simulink model "Alpha_beta_V"  (R2013a)
settings: Solver=ode45  StartTime=0.0  StopTime=10.0  RelTol=1e-3
settings Model: Creator=Ibrahim_B92  LastModifiedBy=Ibrahim_B92

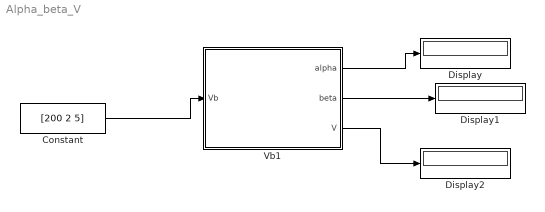
== system Alpha_beta_V ==
  Constant : Constant  Value=[200 2 5]
  Display : Display
  Display1 : Display
  Display2 : Display
  Vb1 : Subsystem
  wires:
  Constant/1 -> Vb1/1(Vb)
  Vb1/1(alpha) -> Display/1
  Vb1/2(beta) -> Display1/1
  Vb1/3(V) -> Display2/1

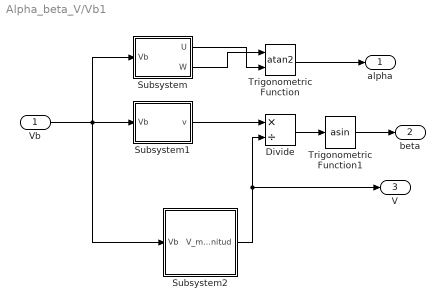
== system Alpha_beta_V/Vb1 ==
  Vb : Inport
  Divide : Product  Inputs=*/
  Subsystem : Subsystem
  Subsystem1 : Subsystem
  Subsystem2 : Subsystem
  Trigonometric Function : Trigonometry  Operator=atan2
  Trigonometric Function1 : Trigonometry  Operator=asin
  alpha : Outport
  beta : Outport  Port=2
  V : Outport  Port=3
  wires:
  Subsystem2/1(V_magnitud) -> Divide/2, V/1
  Subsystem/2(W) -> Trigonometric Function/1
  Subsystem/1(U) -> Trigonometric Function/2
  Trigonometric Function/1 -> alpha/1
  Subsystem1/1(v) -> Divide/1
  Divide/1 -> Trigonometric Function1/1
  Trigonometric Function1/1 -> beta/1
  Vb/1 -> Subsystem2/1(Vb), Subsystem/1(Vb), Subsystem1/1(Vb)

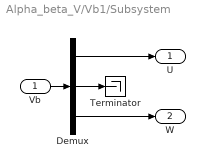
== system Alpha_beta_V/Vb1/Subsystem ==
  Vb : Inport
  Demux : Demux  Outputs=3
  Terminator : Terminator
  U : Outport
  W : Outport  Port=2
  wires:
  Vb/1 -> Demux/1
  Demux/1 -> U/1
  Demux/3 -> W/1
  Demux/2 -> Terminator/1

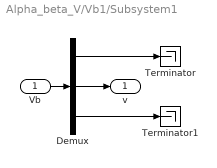
== system Alpha_beta_V/Vb1/Subsystem1 ==
  Vb : Inport
  Demux : Demux  Outputs=3
  Terminator : Terminator
  Terminator1 : Terminator
  v : Outport
  wires:
  Vb/1 -> Demux/1
  Demux/1 -> Terminator/1
  Demux/3 -> Terminator1/1
  Demux/2 -> v/1

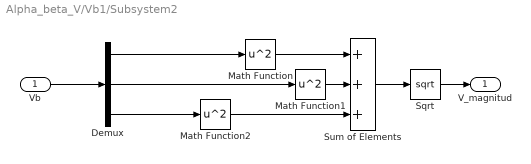
== system Alpha_beta_V/Vb1/Subsystem2 ==
  Vb : Inport
  Demux : Demux  Outputs=3
  Math Function : Math  Operator=square  SaturateOnIntegerOverflow=on
  Math Function1 : Math  Operator=square  SaturateOnIntegerOverflow=on
  Math Function2 : Math  Operator=square  SaturateOnIntegerOverflow=on
  Sqrt : Sqrt  SaturateOnIntegerOverflow=on
  Sum of Elements : Sum  Inputs=+++
  V_magnitud : Outport
  wires:
  Math Function1/1 -> Sum of Elements/2
  Math Function/1 -> Sum of Elements/1
  Math Function2/1 -> Sum of Elements/3
  Sum of Elements/1 -> Sqrt/1
  Sqrt/1 -> V_magnitud/1
  Vb/1 -> Demux/1
  Demux/2 -> Math Function1/1
  Demux/3 -> Math Function2/1
  Demux/1 -> Math Function/1
